simulink model "sim_ICS2026_inv_pendulum"  (R2025b)
settings: Solver=VariableStepAuto  StartTime=0.0  StopTime=Tf  RelTol=1e-3
values from neighbouring files (symbols this model uses):
  A = dt_model.A    [main_Q22_ANN_cart_pend.m]
  Ac = [0, 0, 1, 0 ... (first row only)    [main_Q22_ANN_cart_pend.m]
  add_noise = 1    [main_Q22_ANN_cart_pend.m]
  B = dt_model.B    [main_Q22_ANN_cart_pend.m]
  Bc = [0 ... (first row only)    [main_Q22_ANN_cart_pend.m]
  C = dt_model.C    [main_Q22_ANN_cart_pend.m]
  K_est = [26.6931    2.5463  -12.7832   -3.6866]    [main_Q22_ANN_cart_pend.m]
  Kf_est = [W1'; W2'; W3'; W4']    [main_Q22_ANN_cart_pend.m]
  pos_noise_var = (0.1/100)^2    (= 1e-06)    [main_Q22_ANN_cart_pend.m]
  pos_ref = pi/12    (= 0.261799387799)    [main_Q22_ANN_cart_pend.m]
  ts = 1/1000    (= 0.001)    [main_Q22_ANN_cart_pend.m]
settings Model: Creator=ricardoaguilera  LastModifiedBy=lskje
settings DataIOCC: ReturnWorkspaceOutputs=off
settings DebuggingCC: AlgebraicLoopMsg=none

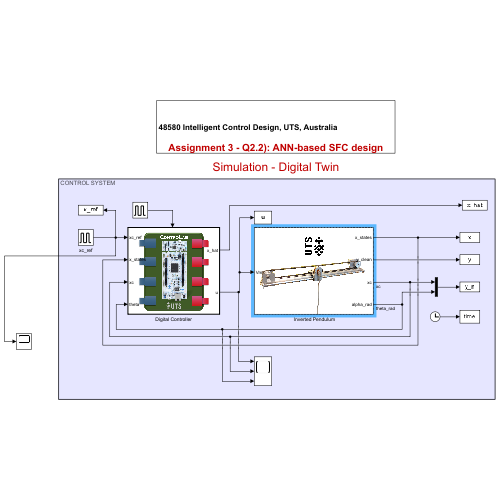
[thumbnail: Simulink's stored preview of the top-level diagram]
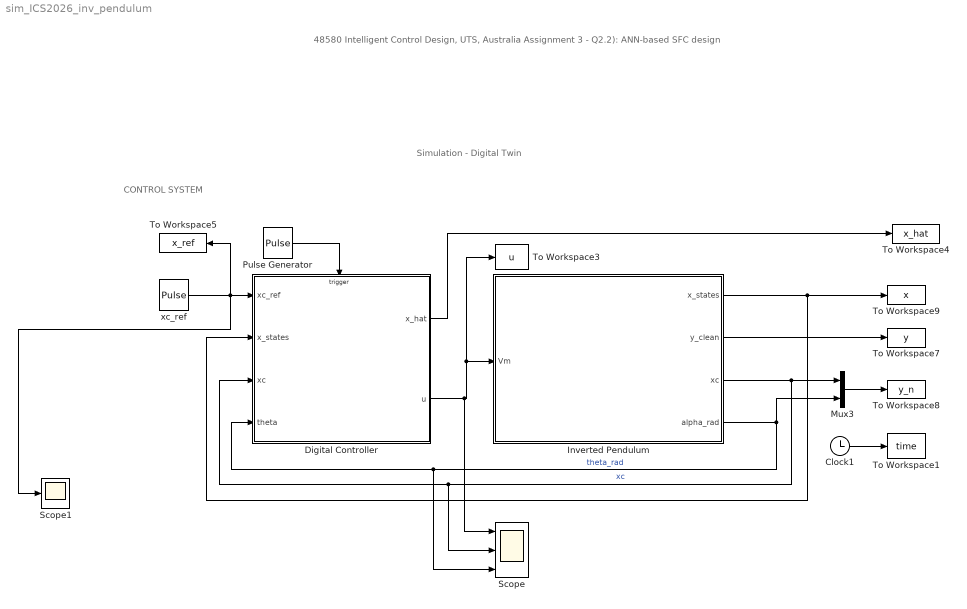
== system sim_ICS2026_inv_pendulum ==
  note: Simulation - Digital Twin
  note: 48580 Intelligent Control Design, UTS, Australia
      |
      | Assignment 3 - Q2.2): ANN-based SFC design
  note: CONTROL SYSTEM
  " Inverted Pendulum" : Subsystem
      mask Display: image('bitmap.png');
  Clock1 : Clock
  Digital Controller : Subsystem  TreatAsAtomicUnit=on
      mask Display: image('Controlboard.png');
  Mux3 : Mux  Inputs=2
  Pulse Generator : DiscretePulseGenerator  PulseType=Time based  Period=ts  PulseWidth=50
  Scope : Scope  NumInputPorts=3
      settings: ActiveDisplayYMinimum=-1  ActiveDisplayYMaximum=1
  Scope1 : Scope
      settings: ActiveDisplayYMinimum=-0.00625  ActiveDisplayYMaximum=0.05625
  To Workspace1 : ToWorkspace  VariableName=time  SampleTime=ts/100
  To Workspace3 : ToWorkspace  VariableName=u  SampleTime=ts/100
  To Workspace4 : ToWorkspace  VariableName=x_hat  SampleTime=ts/100
  To Workspace5 : ToWorkspace  VariableName=x_ref  SampleTime=ts/100
  To Workspace7 : ToWorkspace  VariableName=y  SampleTime=ts/100
  To Workspace8 : ToWorkspace  VariableName=y_n  SampleTime=ts/100
  To Workspace9 : ToWorkspace  VariableName=x  SampleTime=ts/100
  xc_ref : DiscretePulseGenerator  PulseType=Time based  Amplitude=pos_ref  Period=10  PulseWidth=50
  wires:
  Digital Controller/2(u) -> Scope/1, To Workspace3/1, " Inverted Pendulum"/1(Vm)
  Pulse Generator/1 -> Digital Controller/Trigger
  Digital Controller/1(x_hat) -> To Workspace4/1
  xc_ref/1 -> Scope1/1, To Workspace5/1, Digital Controller/1(xc_ref)
  " Inverted Pendulum"/2(y_clean) -> To Workspace7/1
  " Inverted Pendulum"/3(xc) -> Scope/2, Digital Controller/3(xc), Mux3/1  "xc"
  " Inverted Pendulum"/4(alpha_rad) -> Mux3/2, Digital Controller/4(theta), Scope/3  "theta_rad"
  Mux3/1 -> To Workspace8/1
  " Inverted Pendulum"/1(x_states) -> To Workspace9/1, Digital Controller/2(x_states)
  Clock1/1 -> To Workspace1/1

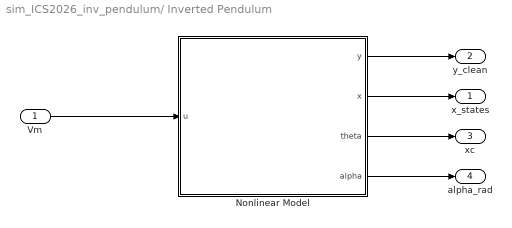
== system sim_ICS2026_inv_pendulum/ Inverted Pendulum ==
  Vm : Inport
  Nonlinear Model : Subsystem
  x_states : Outport
  y_clean : Outport  Port=2
  xc : Outport  Port=3
  alpha_rad : Outport  Port=4
  wires:
  Vm/1 -> Nonlinear Model/1(u)
  Nonlinear Model/3(theta) -> xc/1
  Nonlinear Model/4(alpha) -> alpha_rad/1
  Nonlinear Model/2(x) -> x_states/1
  Nonlinear Model/1(y) -> y_clean/1

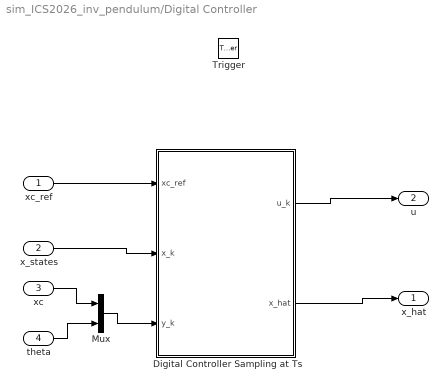
== system sim_ICS2026_inv_pendulum/Digital Controller ==
  xc_ref : Inport
  x_states : Inport  Port=2
  xc : Inport  Port=3
  theta : Inport  Port=4
  Trigger : TriggerPort  VariantControl=(inherit)  InitialTriggerSignalState=zero
  Digital Controller Sampling at Ts : MATLAB Function  TreatAsAtomicUnit=on
  Mux : Mux  Inputs=2
  x_hat : Outport
  u : Outport  Port=2
  wires:
  xc_ref/1 -> Digital Controller Sampling at Ts/1(xc_ref)
  x_states/1 -> Digital Controller Sampling at Ts/2(x_k)
  Digital Controller Sampling at Ts/1(u_k) -> u/1
  xc/1 -> Mux/1
  theta/1 -> Mux/2
  Mux/1 -> Digital Controller Sampling at Ts/3(y_k)
  Digital Controller Sampling at Ts/2(x_hat) -> x_hat/1

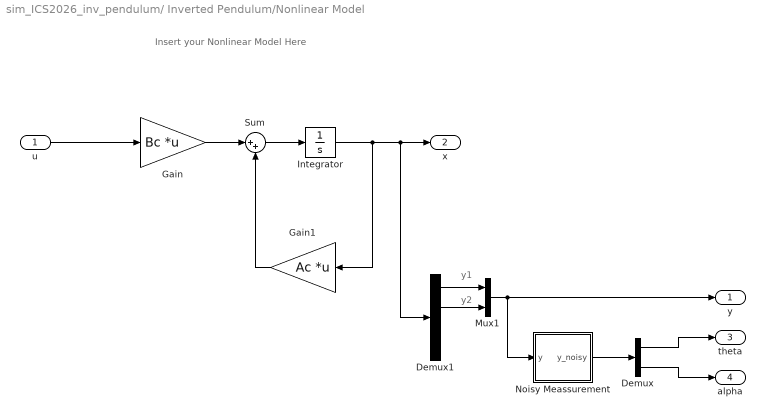
== system sim_ICS2026_inv_pendulum/ Inverted Pendulum/Nonlinear Model ==
  note: Insert your Nonlinear Model Here
  note: y1
  note: y2
  u : Inport
  Demux : Demux  Outputs=2
  Demux1 : Demux
  Gain : Gain  Gain=Bc  Multiplication=Matrix(K*u)
  Gain1 : Gain  Gain=Ac  Multiplication=Matrix(K*u)
  Integrator : Integrator
  Mux1 : Mux  Inputs=2
  Noisy Meassurement : Subsystem
  Sum : Sum  Inputs=|++
  y : Outport  VectorParamsAs1DForOutWhenUnconnected=off
  x : Outport  Port=2  VectorParamsAs1DForOutWhenUnconnected=off
  theta : Outport  Port=3  VectorParamsAs1DForOutWhenUnconnected=off
  alpha : Outport  Port=4  VectorParamsAs1DForOutWhenUnconnected=off
  wires:
  Integrator/1 -> Demux1/1, x/1, Gain1/1
  Mux1/1 -> Noisy Meassurement/1(y), y/1
  Noisy Meassurement/1(y_noisy) -> Demux/1
  Demux/1 -> theta/1
  Demux/2 -> alpha/1
  u/1 -> Gain/1
  Gain1/1 -> Sum/2
  Gain/1 -> Sum/1
  Sum/1 -> Integrator/1
  Demux1/1 -> Mux1/1
  Demux1/2 -> Mux1/2

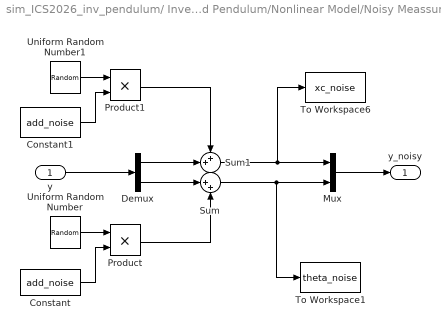
== system sim_ICS2026_inv_pendulum/ Inverted Pendulum/Nonlinear Model/Noisy Meassurement ==
  y : Inport
  Constant : Constant  Value=add_noise
  Constant1 : Constant  Value=add_noise
  Demux : Demux  Outputs=2
  Mux : Mux  Inputs=2
  Product : Product
  Product1 : Product
  Sum : Sum  Inputs=|++
  Sum1 : Sum  Inputs=++|
  To Workspace1 : ToWorkspace  VariableName=theta_noise  SampleTime=ts/100
  To Workspace6 : ToWorkspace  VariableName=xc_noise  SampleTime=ts/100
  Uniform Random Number : UniformRandomNumber  Minimum=-(0.1*pi/180)*1.8  Maximum=(0.1*pi/180)*1.8  Seed=round(rand*10)  SampleTime=ts/10
  Uniform Random Number1 : UniformRandomNumber  Minimum=-sqrt(pos_noise_var)*1.8  Maximum=sqrt(pos_noise_var)*1.8  Seed=round(rand*10)  SampleTime=ts/10
  y_noisy : Outport  VectorParamsAs1DForOutWhenUnconnected=off
  wires:
  Constant1/1 -> Product1/2
  y/1 -> Demux/1
  Mux/1 -> y_noisy/1
  Demux/1 -> Sum1/2
  Product1/1 -> Sum1/1
  Demux/2 -> Sum/1
  Product/1 -> Sum/2
  Sum1/1 -> To Workspace6/1, Mux/1
  Sum/1 -> To Workspace1/1, Mux/2
  Constant/1 -> Product/2
  Uniform Random Number/1 -> Product/1
  Uniform Random Number1/1 -> Product1/1

== matlab function sim_ICS2026_inv_pendulum/Digital Controller/Digital Controller Sampling at Ts ==
  data: xc_ref input; x_k input; u_k output; K_est parameter; y_k input; x_hat output; A parameter; B parameter; C parameter; Kf_est parameter
function [u_k,x_hat] = fcn(xc_ref,x_k,K_est, y_k, A, B, C, Kf_est)

%% Observer
persistent x_hat_prev u_prev
if isempty(x_hat_prev)
   x_hat_prev = [0 0 0 0]';
   u_prev = 0;
end

x_hat = A*x_hat_prev + B*u_prev + Kf_est*(y_k-C*x_hat_prev);

%% SFC

u_k = -K_est*(x_hat - xc_ref*[1 0 0 0]');

u_prev = u_k;
x_hat_prev = x_hat;
